simulink model "feng_ct"  (R2016b)
(part 3 of 81)

      | port_label('output', 1, 'q');
      | disp(['Z^-', num2str(latency)]);
  we_delay95 : Subsystem  AncestorBlock=casper_library_delays/pipeline  mask(pipeline){latency=5}
      mask help:
      | An explicitly laid-out delay line to avoid mapping to SRL16s
      | for use in pipelining to help achieve timing closure.
      mask init:
      | pipeline_init(gcb,'latency',latency);
      settings: AttributesFormatString=Latency = %<latency>
      mask Display:
      | port_label('input', 1, 'd');
      | port_label('output', 1, 'q');
      | disp(['Z^-', num2str(latency)]);
  we_delay96 : Subsystem  AncestorBlock=casper_library_delays/pipeline  mask(pipeline){latency=3}
      mask help:
      | An explicitly laid-out delay line to avoid mapping to SRL16s
      | for use in pipelining to help achieve timing closure.
      mask init:
      | pipeline_init(gcb,'latency',latency);
      settings: AttributesFormatString=Latency = %<latency>
      mask Display:
      | port_label('input', 1, 'd');
      | port_label('output', 1, 'q');
      | disp(['Z^-', num2str(latency)]);
  we_delay97 : Subsystem  AncestorBlock=casper_library_delays/pipeline  mask(pipeline){latency=5}
      mask help:
      | An explicitly laid-out delay line to avoid mapping to SRL16s
      | for use in pipelining to help achieve timing closure.
      mask init:
      | pipeline_init(gcb,'latency',latency);
      settings: AttributesFormatString=Latency = %<latency>
      mask Display:
      | port_label('input', 1, 'd');
      | port_label('output', 1, 'q');
      | disp(['Z^-', num2str(latency)]);
  we_delay98 : Subsystem  AncestorBlock=casper_library_delays/pipeline  mask(pipeline){latency=5}
      mask help:
      | An explicitly laid-out delay line to avoid mapping to SRL16s
      | for use in pipelining to help achieve timing closure.
      mask init:
      | pipeline_init(gcb,'latency',latency);
      settings: AttributesFormatString=Latency = %<latency>
      mask Display:
      | port_label('input', 1, 'd');
      | port_label('output', 1, 'q');
      | disp(['Z^-', num2str(latency)]);
  we_delay99 : Subsystem  AncestorBlock=casper_library_delays/pipeline  mask(pipeline){latency=3}
      mask help:
      | An explicitly laid-out delay line to avoid mapping to SRL16s
      | for use in pipelining to help achieve timing closure.
      mask init:
      | pipeline_init(gcb,'latency',latency);
      settings: AttributesFormatString=Latency = %<latency>
      mask Display:
      | port_label('input', 1, 'd');
      | port_label('output', 1, 'q');
      | disp(['Z^-', num2str(latency)]);
  xsg_core_config : Subsystem  Tag=xps:xsg  AncestorBlock=xps_library/XSG_core_config  mask(xsg core config){hw_sys=SKARAB:xc7vx690t, clk_src=sys_clk, clk_rate=238, sample_period=1, synthesis_tool=XST}
      mask prompts: hw_sys "Hardware Platform"; clk_src "User IP Clock source"; clk_rate "User IP Clock Rate (MHz)"; sample_period "Sample Period"; synthesis_tool "Synthesis Tool:"
      mask help:
      | The XSG Core Config block is used to configure the System Generator design
      | for the casper_xps toolflow. Settings here are used to configure the
      | Xilinx System Generator block parameters automatically, and control toolflow
      | script  execution. It needs to be at the top level of all designs being compiled
      | with the casper_xps toolflow.
      mask init:
      | xps_xsg_conf_mask;
      mask Help: eval('xlWeb([getenv(''MLIB_ROOT''), ''\doc\html\sys_xsg_core_config\sys_xsg_core_config.html''])')
      mask TypeOptions hw_sys: ROACH:sx95t | ROACH:lx110t | ROACH2:sx475t | SNAP:xc7k160t | KC705:xc7k325t | SKARAB:xc7vx690t
      mask Callback hw_sys: xps_xsg_conf_callback
      mask TypeOptions clk_src: sys_clk | aux_clk
      mask Callback clk_src: xps_xsg_conf_callback
      mask Callback clk_rate: xps_xsg_conf_callback
      mask TypeOptions synthesis_tool: Leonardo Spectrum | Synplify | Synplify Pro | XST
      mask Display: fprintf(['MSSGE\n', hw_sys]);
  tag scope: cnt_rst=global, ct_chans_per_board=global, ct_chans_per_x=global, ct_chans_per_x_hmc_par=global, ct_chans_per_x_hmc_par_recip=global, ct_chans_per_x_par=global, ct_chans_per_x_recip=global, ct_fake_data_error=global, ct_num_x_boards=global, ct_num_x_boards_recip=global, ct_num_xeng=global, ct_num_xeng_recip=global, ct_rst_err_latch=global, ct_tag_insert_sel=global, ct_tvg_en2=global, ct_tvg_en=global, ct_x_per_board=global, ct_x_per_board_recip=global, obuf_read_gap=global, pktoffset_sel=global, pktstart_sel=global, sys_rst=global, tvgtone_levels=global, tvgtone_p0=global, tvgtone_p1=global, up_timestep_error=global
  wires:
  Constant3/1 -> gbe0/8(rx_overrun_ack)
  Constant4/1 -> gbe0/7(rx_ack)
  [gbe_rst] -> pipeline99/1(d)
  unpack_and_reorder/5(recvd) -> pipeline17/1(d)
  sync_gen/2(dout) -> bus_expand6/1(bus_in)
  sync_gen/3(dvalid) -> impulse_gen0/6(en), impulse_gen1/6(en)
  Slice4/1 -> pipeline16/1(d)
  pipeline16/1(q) -> local_time_lsw/1(out_timestamp_lsw)
  Slice16/1 -> Convert6/1
  pipeline47/1(q) -> local_time_msw/1(out_timestamp_msw)
  Convert6/1 -> pipeline47/1(d)
  [time80_48] -> Slice16/1, Slice4/1
  Concat22/1 -> [ld_val0]
  Concat3/1 -> [ld_val1]
  bus_expand17/1(msb_out2) -> [unpack_recvd0]
  bus_expand17/2(lsb_out1) -> [unpack_recvd1]
  Slice12/1 -> [time80]
  impulse_gen0/3(dvalid) -> [valid80]
  impulse_gen0/1(sync_out) -> [sync80]
  impulse_gen0/2(dout) -> [d80_adc0]
  impulse_gen0/4(misco) -> [time80_48], Slice12/1
  [tvg_adc_en] -> impulse_gen0/1(tvg_en)
  impulse_gen1/1(sync_out) -> Terminator6/1
  impulse_gen1/2(dout) -> [d80_adc1]
  impulse_gen1/3(dvalid) -> Terminator8/1
  impulse_gen1/4(misco) -> [dig_flags]
  [tvg_adc_en] -> impulse_gen1/1(tvg_en)
  impulse0/1(in_offset) -> Slice7/1
  impulse0/2(in_amplitude) -> impulse_gen0/3(impulse_amplitude)
  impulse1/1(in_offset) -> Slice8/1
  impulse1/2(in_amplitude) -> impulse_gen1/3(impulse_amplitude)
  sync_gen/1(sync) -> impulse_gen0/4(sync_in), impulse_gen1/4(sync_in)
  bus_expand6/1(msb_out2) -> impulse_gen0/5(din)
  bus_expand6/2(lsb_out1) -> impulse_gen1/5(din)
  sync_gen/5(misco) -> impulse_gen1/7(misci)
  sync_gen/4(time_out) -> impulse_gen0/7(misci)
  Constant31/1 -> Concat9/2
  [unpack_timestamp] -> Concat9/1
  [up_timestep_error] -> Logical15/1
  [sys_rst] -> Logical15/2
  Logical15/1 -> edge_detect17/1(in)
  edge_detect17/1(out) -> [sys_relock]
  phase0/1(in_initial) -> Reinterpret2/1
  delta_delay0/1(in_delta) -> Reinterpret1/1
  phase0/2(in_delta) -> Reinterpret3/1
  Concat9/1 -> sync_gen/1(time_in)
  [sys_relock] -> sync_gen/5(relock)
  [unpack_dv] -> sync_gen/2(en)
  [unpack_d160] -> sync_gen/3(din)
  Slice7/1 -> impulse_gen0/2(impulse_offset)
  Slice8/1 -> impulse_gen1/2(impulse_offset)
  Reinterpret8/1 -> Concat22/1
  Reinterpret1/1 -> Concat22/2
  Reinterpret2/1 -> Concat22/3
  Reinterpret3/1 -> Concat22/4
  phase1/1(in_initial) -> Reinterpret5/1
  delta_delay1/1(in_delta) -> Reinterpret4/1
  phase1/2(in_delta) -> Reinterpret6/1
  Reinterpret4/1 -> Concat3/2
  Reinterpret5/1 -> Concat3/3
  Reinterpret6/1 -> Concat3/4
  Reinterpret7/1 -> Concat3/1
  delay0/1(in_initial) -> Reinterpret8/1
  delay1/1(in_initial) -> Reinterpret7/1
  trig_time_msw/1(in_msw) -> pipeline28/1(d)
  trig_time_lsw/1(in_lsw) -> pipeline44/1(d)
  Concat13/1 -> Relational10/1
  pipeline28/1(q) -> Concat13/1
  pipeline44/1(q) -> Concat13/2
  [valid80] -> Counter/2
  [sync80] -> Counter/1
  Constant12/1 -> Relational7/2
  Counter/1 -> Relational7/1
  Relational10/1 -> Mux/2
  Relational7/1 -> Mux/3
  [valid80] -> Delay49/1
  Logical12/1 -> Logical14/1
  Logical14/1 -> [adc_snap_trig]
  [adc_snap_arm] -> Logical14/2
  [time80_48] -> Relational10/2
  Delay49/1 -> Logical12/2
  Mux/1 -> Logical12/1
  [adc_snap_trig_source] -> Mux/1
  iptx_base/1(in_reg) -> pipeline105/1(d)
  pipeline105/1(q) -> [tx_ip_base]
  tx_metadata/1(in_porttx) -> pipeline106/1(d)
  tx_metadata/2(in_board_id) -> pipeline107/1(d)
  pipeline106/1(q) -> [tx_port]
  pipeline107/1(q) -> changing_bits2/1
  edge_detect4/1(out) -> pipeline5/1(d)
  control/6(in_cnt_rst) -> edge_detect1/1(in)
  edge_detect1/1(out) -> pipeline14/1(d)
  control/3(in_gbe_rst) -> pipeline6/1(d)
  control/1(in_sys_rst) -> pipeline3/1(d)
  pipeline3/1(q) -> [sys_rst]
  pipeline5/1(q) -> [clr_status]
  pipeline6/1(q) -> [gbe_rst]
  pipeline7/1(q) -> [gbe_txen]
  pipeline13/1(q) -> [tvg_adc_en]
  pipeline14/1(q) -> [cnt_rst]
  control/5(in_tvg_adc) -> pipeline13/1(d)
  edge_detect2/1(out) -> pipeline38/1(d)
  pipeline38/1(q) -> [gbe_cnt_rst]
  control/7(in_gbe_cnt_rst) -> edge_detect2/1(in)
  control/4(in_gbe_txen) -> pipeline7/1(d)
  control/2(in_status_clr) -> edge_detect4/1(in)
  pipeline43/1(q) -> [adc_snap_arm]
  control/8(in_adc_snap_arm) -> pipeline43/1(d)
  control/9(in_adc_snap_trig_select) -> pipeline39/1(d)
  pipeline39/1(q) -> [adc_snap_trig_source]
  pfb/2(dout0) -> [pfb_d144_0]
  pfb/3(dout1) -> [pfb_d144_1]
  [fft_shift] -> pfb/1(shift)
  fft_shift/1(in_fft_shift) -> pipeline4/1(d)
  pfb/5(of) -> [pfb_of]
  pfb/4(dvalid) -> [pfb_dv]
  pfb/1(sync_out) -> [pfb_sync]
  [pfbin_d1] -> pfb/4(din1)
  [pfbin_d0] -> pfb/3(din0)
  [pfbin_sync] -> pfb/2(sync_in)
  [pfbin_dv] -> pfb/5(en)
  tl_fd0/2(enable) -> phase_compensation0/5(load_value)
  tl_fd1/1(value) -> phase_compensation1/4(delay_value)
  tl_fd1/2(enable) -> phase_compensation1/5(load_value)
  tl_fd0/1(value) -> phase_compensation0/4(delay_value)
  [clr_status] -> tl_fd1/1(rst), tl_fd0/1(rst)
  phase_compensation0/1(sync_out) -> [fdfs_sync]
  phase_compensation1/1(sync_out) -> Terminator24/1
  phase_compensation0/2(dout) -> [fdfs_d144_0]
  phase_compensation1/2(dout) -> [fdfs_d144_1]
  phase_compensation0/3(dvalid) -> [fdfs_dv]
  phase_compensation1/3(dvalid) -> Terminator25/1
  [ld_val0] -> tl_fd0/3(load_value)
  [ld_val1] -> tl_fd1/3(load_value)
  bus_expand16/1(msb_out2) -> tl_fd0/5(din)
  tl_fd0/5(dvalid) -> phase_compensation0/3(en)
  tl_fd0/3(sync_out) -> phase_compensation0/1(sync_in)
  tl_fd0/4(dout) -> phase_compensation0/2(din)
  tl_fd1/4(dout) -> phase_compensation1/2(din)
  bus_expand16/2(lsb_out1) -> tl_fd1/5(din)
  Constant29/1 -> Concat2/2
  Concat2/1 -> tl_fd1/2(current_time), tl_fd0/2(current_time)
  [gbe_cnt_rst] -> pipeline31/1(d)
  pipeline31/1(q) -> gbe0/9(debug_rst)
  Counter2/1 -> pipeline29/1(d)
  Constant26/1 -> eq1/2(data_in)
  Constant11/1 -> eq1/3(we)
  Delay53/1 -> quant1/1(sync_in)
  Delay34/1 -> quant1/2(din)
  eq1/1(data_out) -> quant1/4(coeffs)
  Delay50/1 -> quant1/3(en)
  Counter4/1 -> pipeline27/1(d)
  Constant24/1 -> eq0/2(data_in)
  Constant25/1 -> eq0/3(we)
  Delay51/1 -> quant0/1(sync_in)
  Delay2/1 -> quant0/2(din)
  Delay52/1 -> quant0/3(en)
  eq0/1(data_out) -> quant0/4(coeffs)
  quant0/1(sync_out) -> [q_sync]
  quant0/2(dout) -> Delay7/1
  quant0/3(dvalid) -> Delay6/1
  quant0/4(of) -> Delay11/1
  quant1/2(dout) -> Delay12/1
  quant1/1(sync_out) -> Terminator19/1
  quant1/3(dvalid) -> Terminator21/1
  quant1/4(of) -> Delay13/1
  pipeline27/1(q) -> eq0/1(addr)
  pipeline29/1(q) -> eq1/1(addr)
  [fdfs_sync] -> Delay51/1, pipeline42/1(d)
  [fdfs_d144_0] -> Delay2/1
  [fdfs_dv] -> Delay52/1, pipeline41/1(d)
  pipeline41/1(q) -> Counter4/2
  pipeline42/1(q) -> Counter4/1
  pipeline45/1(q) -> Counter2/2
  [fdfs_sync] -> Delay53/1, pipeline48/1(d)
  [fdfs_d144_1] -> Delay34/1
  [fdfs_dv] -> Delay50/1, pipeline45/1(d)
  pipeline48/1(q) -> Counter2/1
  gbe0/13(rx_dest_ip) -> pipeline115/1(d)
  gbe0/14(rx_dest_port) -> pipeline116/1(d)
  [rx_dest_ip] -> pipeline/1(d)
  pipeline/1(q) -> rx_dest_ip/1(out_reg)
  [rx_dest_port] -> pipeline18/1(d)
  pipeline18/1(q) -> rx_dest_port/1(out_reg)
  gbe0/1(led_up) -> pipeline100/1(d)
  [forty_gbe_led_up] -> pipeline19/1(d)
  gbe0/2(led_rx) -> pipeline101/1(d)
  [forty_gbe_led_rx] -> pipeline20/1(d)
  gbe0/3(led_tx) -> pipeline102/1(d)
  [forty_gbe_led_tx] -> pipeline51/1(d)
  gbe0/4(tx_afull) -> pipeline103/1(d)
  gbe0/5(tx_overflow) -> pipeline104/1(d)
  gbe0/12(rx_overrun) -> pipeline114/1(d)
  pipeline19/1(q) -> gbe_status/1(out_led_up)
  pipeline20/1(q) -> gbe_status/2(out_led_rx)
  pipeline51/1(q) -> gbe_status/3(out_led_tx)
  gbe0/8(rx_source_ip) -> pipeline110/1(d)
  gbe0/9(rx_source_port) -> pipeline111/1(d)
  pipeline55/1(q) -> rx_src_ip/1(out_reg)
  pipeline56/1(q) -> rx_src_port/1(out_reg)
  [forty_gbe_rx_src_port] -> pipeline56/1(d)
  [forty_gbe_rx_src_ip] -> pipeline55/1(d)
  gbe0/6(rx_data) -> pipeline108/1(d)
  gbe0/10(rx_end_of_frame) -> pipeline112/1(d)
  gbe0/11(rx_bad_frame) -> pipeline113/1(d)
  pipeline174/1(q) -> time_gen1/5(rd_en)
  pipeline173/1(q) -> time_gen1/4(rd_sync_in)
  pipeline80/1(q) -> [flag_sync]
  pipeline81/1(q) -> [flag_misc]
  pipeline82/1(q) -> [flag_dvalid]
  pipeline83/1(q) -> [flag_time]
  [s256_d] -> pipeline98/1(d)
  [s256_ip] -> pipeline97/1(d)
  [s256_port] -> pipeline96/1(d)
  Logical2/1 -> gbe0/6(tx_end_of_frame)
  [s256_v] -> Logical1/2
  [s256_eof] -> Logical2/2
  Delay1/1 -> Logical1/1, Logical2/1
  [s256_eof] -> Delay1/2
  pipeline96/1(q) -> gbe0/5(tx_dest_port)
  pipeline97/1(q) -> gbe0/4(tx_dest_ip)
  pipeline98/1(q) -> gbe0/2(tx_data)
  pipeline99/1(q) -> gbe0/1(rst)
  [gbe_txen] -> Delay1/1
  pipeline100/1(q) -> [forty_gbe_led_up]
  pipeline101/1(q) -> [forty_gbe_led_rx]
  pipeline102/1(q) -> [forty_gbe_led_tx]
  pipeline103/1(q) -> [forty_gbe_tx_full]
  pipeline104/1(q) -> [forty_gbe_tx_of]
  pipeline108/1(q) -> [forty_gbe_rx_data]
  pipeline110/1(q) -> [forty_gbe_rx_src_ip]
  pipeline111/1(q) -> [forty_gbe_rx_src_port]
  pipeline112/1(q) -> [forty_gbe_rx_eof]
  pipeline113/1(q) -> [forty_gbe_rx_bad]
  pipeline114/1(q) -> [forty_gbe_rx_overrun]
  pipeline115/1(q) -> [rx_dest_ip]
  pipeline116/1(q) -> [rx_dest_port]
  [forty_gbe_rx_data] -> unpack_and_reorder/1(d256)
  [forty_gbe_rx_valid] -> unpack_and_reorder/2(dv256)
  [forty_gbe_rx_eof] -> unpack_and_reorder/3(eof256)
  unpack_and_reorder/6(flags) -> Terminator9/1
  unpack_and_reorder/2(d160) -> pipeline11/1(d)
  unpack_and_reorder/3(dv) -> pipeline12/1(d)
  unpack_and_reorder/4(time) -> pipeline15/1(d)
  unpack_and_reorder/1(sync) -> pipeline10/1(d)
  Inverter1/1 -> Logical6/1
  [unpack_recvd0] -> Inverter1/1
  [unpack_dv] -> Logical6/2
  Inverter2/1 -> Logical7/1
  [unpack_recvd1] -> Inverter2/1
  [unpack_dv] -> Logical7/2
  Logical7/1 -> Logical/2
  Logical6/1 -> Logical/1
  Logical/1 -> [unpack_missing]
  pipeline10/1(q) -> [unpack_sync]
  pipeline11/1(q) -> [unpack_d160]
  pipeline12/1(q) -> [unpack_dv]
  pipeline15/1(q) -> [unpack_timestamp]
  pipeline17/1(q) -> bus_expand17/1(bus_in)
  [clr_status] -> Counter1/1, Subsystem5/1(rst)
  [up_dbg_rst] -> Subsystem4/1(rst)
  [upg_sp_dv] -> Logical3/2
  [upg_sp_eof] -> Logical3/1
  [upg_reo_time] -> Subsystem1/3(time)
  [upg_reo_recv] -> Subsystem1/4(recv)
  [upg_reo_dv] -> Subsystem7/1(dv), Subsystem1/2(dv)
  [up_dbg_rst] -> Subsystem1/1(rst)
  Subsystem1/7(time_change) -> [reo_time_change]
  Logical5/1 -> Subsystem1/7(overflow_err)
  [upg_of80_p1] -> Logical5/2
  [upg_of80_p0] -> Logical5/1
  [upg_sperr_magic] -> Subsystem4/2(in0)
  [upg_sperr_len] -> Subsystem4/5(in3)
  [upg_sperr_hdr] -> Subsystem4/3(in1)
  [upg_sperr_pad] -> Subsystem4/4(in2)
  pipeline175/1(q) -> time_gen1/6(rd_misc_in)
  tl_fd0/7(misco) -> Terminator2/1
  tl_fd0/6(time) -> Terminator3/1
  tl_fd1/6(time) -> Terminator4/1
  tl_fd1/3(sync_out) -> phase_compensation1/1(sync_in)
  tl_fd1/5(dvalid) -> phase_compensation1/3(en)
  tl_fd1/7(misco) -> Terminator5/1
  Constant18/1 -> tl_fd0/7(misci)
  Constant19/1 -> tl_fd1/7(misci)
  Subsystem4/5(out4) -> spead_status/5(out_pkt_cnt)
  Logical3/1 -> Subsystem4/6(in4)
  Constant1/1 -> sync_gen/4(misci)
  time_gen/1(rd_sync_out) -> tl_fd1/4(sync_in), tl_fd0/4(sync_in)
  time_gen/2(rd_dvalid) -> tl_fd1/6(en), tl_fd0/6(en)
  time_gen/3(rd_val_out) -> Concat2/1
  time_gen/4(rd_misc_out) -> bus_expand16/1(bus_in)
  [sync80] -> time_gen/1(wr_sync_in)
  [valid80] -> time_gen/2(wr_en)
  [pfb_sync] -> time_gen/4(rd_sync_in)
  [pfb_dv] -> time_gen/5(rd_en)
  [pfb_d144_1] -> Concat1/2
  [pfb_d144_0] -> Concat1/1
  Concat1/1 -> time_gen/6(rd_misc_in)
  [q_sync] -> time_gen1/1(wr_sync_in)
  [q_dv] -> time_gen1/2(wr_en)
  [time80] -> Slice2/1
  time_gen1/1(rd_sync_out) -> pipeline80/1(d)
  time_gen1/4(rd_misc_out) -> pipeline81/1(d)
  time_gen1/2(rd_dvalid) -> pipeline82/1(d)
  time_gen1/3(rd_val_out) -> pipeline83/1(d)
  [time80] -> time_gen/3(wr_val_in)
  Slice2/1 -> time_gen1/3(wr_val_in)
  pipeline4/1(q) -> [fft_shift]
  Logical1/1 -> gbe0/3(tx_valid)
  pipeline59/1(q) -> [ct_tvg_en]
  control/10(in_ct_tvg_en) -> pipeline59/1(d)
  pipeline52/1(q) -> [up_dbg_rst]
  control/11(in_unpack_debug_reset) -> pipeline52/1(d)
  Subsystem1/8(timestep_err) -> [up_timestep_error]
  Subsystem4/4(out3) -> spead_status/4(out_pkt_len_err_cnt)
  Subsystem4/3(out2) -> spead_status/3(out_pad_err_cnt)
  Subsystem4/2(out1) -> spead_status/2(out_header_err_cnt)
  Subsystem4/1(out0) -> spead_status/1(out_magic_err_cnt)
  [upg_reo_disc] -> Subsystem1/5(discard_err)
  [upg_reo_relock] -> Subsystem1/6(relock_err)
  Subsystem1/1(timestep_err_cnt) -> reorder_status/1(out_timestep_err_cnt)
  Subsystem1/2(recv_err_cnt) -> reorder_status/2(out_receive_err_cnt)
  Subsystem1/3(discard_err_cnt) -> reorder_status/3(out_discard_cnt)
  Subsystem1/4(relock_err_cnt) -> reorder_status/4(out_relock_err_cnt)
  Subsystem1/5(overflow_err_cnt) -> reorder_status/5(out_overflow_err_cnt)
  Subsystem2/1(out0) -> cd_status/1(out_hmc_err_cnt)
  Subsystem2/2(out1) -> cd_status/2(out_pol0_parity_err_cnt)
  Subsystem2/3(out2) -> cd_status/3(out_pol1_parity_err_cnt)
  [hmc_parity_pol0] -> Subsystem2/3(in1)
  [hmc_parity_pol1] -> Subsystem2/4(in2)
  [clr_status] -> Subsystem2/1(rst)
  [hmc_error] -> Subsystem2/2(in0)
  [clr_status] -> Subsystem3/1(rst)
  Slice/1 -> Subsystem3/2(in0)
  [pfb_of] -> Slice/1, Slice6/1
  Slice6/1 -> Subsystem3/3(in1)
  [pfb_sync] -> Subsystem3/4(in2)
  Subsystem3/3(out2) -> pfb_status/3(out_sync_cnt)
  Subsystem5/1(out0) -> quant_status/1(out_pol0_or_cnt)
  Relational/1 -> Subsystem5/2(in0)
  Constant10/1 -> Relational/2
  [q_of0] -> Relational/1
  Relational3/1 -> Subsystem5/3(in1)
  [q_of1] -> Relational3/1
  Constant13/1 -> Relational3/2
  Subsystem5/2(out1) -> quant_status/2(out_pol1_or_cnt)
  Subsystem3/1(out0) -> pfb_status/1(out_pol0_or_err_cnt)
  Subsystem3/2(out1) -> pfb_status/2(out_pol1_or_err_cnt)
  [q_sync] -> hmc_ct/1(in_sync)
  [q_d64_1] -> Concat4/1
  [q_d64_0] -> Concat4/2
  hmc_ct/4(pkt_start) -> [ct_pktstart]
  [ct_tvg_en2] -> Mux1/1
  hmc_ct/1(out_sync) -> [ct_sync]
  hmc_ct/2(out_dv) -> [ct_dv]
  hmc_ct/3(out_d256) -> [ct_d256]
  [ct_dv] -> pipeline86/1(d)
  pipeline87/1(q) -> Mux1/2
  pipeline85/1(q) -> tvg/1(sync), pipeline89/1(d)
  [ct_sync] -> pipeline85/1(d)
  [ct_d256] -> pipeline87/1(d)
  pipeline89/1(q) -> pipeline173/1(d)
  pipeline88/1(q) -> pipeline174/1(d)
  Mux1/1 -> pipeline175/1(d)
  pipeline86/1(q) -> tvg/2(dv), pipeline88/1(d)
  Subsystem1/6(dv_cnt) -> reorder_status/6(out_dv_cnt)
  [flag_dvalid] -> Subsystem13/1(In1)
  Subsystem13/1(Out1) -> time_status/1(out_dv_cnt)
  tvg/1(data256) -> Mux1/3
  [ct_dv] -> Subsystem8/1(In1)
  Subsystem8/1(Out1) -> ct_dv_rate/1(out_reg)
  we_delay49/1(q) -> [ct_tag_insert_sel]
  edge_detect3/1 -> [ct_rst_err_latch]
  we_delay47/1(q) -> edge_detect3/1
  we_delay48/1(q) -> [ct_fake_data_error]
  we_delay13/1(q) -> [ct_tvg_en]
  we_delay50/1(q) -> [ct_tvg_en2]
  Constant2/1 -> ct_control0/5(sim_5)
  Constant21/1 -> ct_control0/4(sim_4)
  Constant20/1 -> ct_control0/3(sim_3)
  Constant22/1 -> ct_control0/2(sim_2)
  Constant15/1 -> ct_control0/1(sim_1)
  ct_control0/1(in_tvg_en) -> we_delay13/1(d)
  ct_control0/2(in_tvg_en2) -> we_delay50/1(d)
  ct_control0/3(in_rst_err_latch) -> we_delay47/1(d)
  ct_control0/4(in_fake_error) -> we_delay48/1(d)
  ct_control0/5(in_tag_insert) -> we_delay49/1(d)
  pipeline75/1(q) -> pipeline62/1(d)
  [gbe_stopmux] -> multimux4/1(select)
  [forty_gbe_tx_of] -> multimux4/2(input1)
  [forty_gbe_tx_full] -> multimux4/3(input2)
  [forty_gbe_tx_err] -> multimux4/4(input3)
  [q_sync] -> edge_detect/1
  edge_detect/1 -> Counter1/2
  Counter1/1 -> quant_status/3(out_sync_cnt)
  [ct_pktstart] -> we_delay1/1(d)
  [ct_dv] -> we_delay2/1(d)
  we_delay1/1(q) -> pktlen_check/1(pkt_start)
  we_delay2/1(q) -> dv_block_check/1(dv), pktlen_check/2(dv)
  pktlen_check/1(error) -> we_delay7/1(d)
  dv_block_check/1(error) -> we_delay29/1(d)
  [cnt_rst] -> Subsystem6/1(rst)
  we_delay7/1(q) -> [ct_pktlen_err], Subsystem6/2(in0)
  we_delay29/1(q) -> [ct_dvblk_err], Subsystem6/3(in1)
  Subsystem6/1(out0) -> ct_dv_err/1(out_pktlen_err_cnt)
  Subsystem6/2(out1) -> ct_dv_err/2(out_dvblock_err_cnt)
  [q_dv] -> qt_block_check/1(dv)
  [cnt_rst] -> Subsystem12/1(rst)
  Subsystem12/1(out0) -> qt_dv_err/1(out_dvblock_err_cnt)
  [pack_dv_err] -> multimux4/5(input4)
  [unpack_dv] -> reo_block_check/1(dv)
  [cnt_rst] -> Subsystem15/1(rst)
  Subsystem15/1(out0) -> reo_dv_err/1(out_dvblock_err_cnt)
  reo_block_check/1(error) -> Subsystem15/2(in0)
  [sync80] -> Mux4/2
  [cd_bypass] -> Mux4/1
  [delay_sync] -> Mux4/3
  [valid80] -> Mux5/2
  [cd_bypass] -> Mux5/1
  [delay_dv] -> Mux5/3
  Mux4/1 -> [pfbin_sync]
  Mux5/1 -> [pfbin_dv]
  [d80_adc0] -> Mux6/2
  [cd_bypass] -> Mux6/1
  [delay_d0] -> Mux6/3
  Mux6/1 -> [pfbin_d0]
  [d80_adc1] -> Mux7/2
  [cd_bypass] -> Mux7/1
  [delay_d1] -> Mux7/3
  Mux7/1 -> [pfbin_d1]
  pipeline57/1(q) -> [cd_bypass]
  control/12(in_cd_bypass) -> pipeline57/1(d)
  Constant7/1 -> [delay_sync]
  Constant23/1 -> [delay_d0]
  Constant27/1 -> [delay_dv]
  Constant37/1 -> [delay_d1]
  Constant40/1 -> [hmc_error]
  Constant39/1 -> [hmc_parity_pol0]
  Constant38/1 -> [hmc_parity_pol1]
  [cnt_rst] -> Subsystem17/1(rst)
  Subsystem17/1(out0) -> ct_dout_err0/1(out_pol_error_cnt)
  Subsystem17/2(out1) -> ct_dout_err0/2(out_word_error_cnt)
  pktlen_check2/1(error) -> [ct_tvg_data_order_err]
  Subsystem17/3(out2) -> ct_dout_err0/3(out_dout_order_err)
  Register2/1 -> Relational20/2
  [ct_dv] -> Relational20/3, Register2/2  "dv"
  Relational20/1 -> pktlen_check2/1(pkt_start)  "newdata"
  Delay9/1 -> pktlen_check2/2(dv)  "dv_del"
  [ct_dv] -> Delay9/1
  Slice35/1 -> Relational20/1, Register2/1
  [cnt_rst] -> Subsystem9/1(rst)
  [ct_bank_error_g0] -> Subsystem9/2(in0)
  [ct_en_sync_error_g0] -> Subsystem9/3(in1)
  [wr_data_final_g0] -> bus_expand5/1(bus_in)
  bus_expand5/1(msb_out16) -> Slice30/1
  bus_expand5/2(out15) -> Slice25/1
  bus_expand5/3(out14) -> Slice13/1
  bus_expand5/4(out13) -> Slice26/1
  bus_expand5/9(out8) -> Slice24/1
  bus_expand5/10(out7) -> Slice14/1
  bus_expand5/11(out6) -> Slice15/1
  bus_expand5/12(out5) -> Slice22/1
  Slice30/1 -> [rawd0_0]
  Slice25/1 -> [rawd1_0]
  Slice13/1 -> [rawd2_0]
  Slice26/1 -> [rawd3_0]
  Slice22/1 -> [rawd7_0]
  Slice15/1 -> [rawd6_0]
  Slice14/1 -> [rawd5_0]
  Slice24/1 -> [rawd4_0]
  [ct_pktlen_err] -> Logical22/1
  [ct_dvblk_err] -> Logical22/2
  Logical22/1 -> multimux1/2(input1)
  [wrrd_stopmux] -> Slice44/1
  [ct_tvg_data_order_err] -> multimux1/3(input2)
  [ct_snap_err_stop] -> Logical22/3
  [rawd1_0] -> data_repeat_error/1(data)
  [wr_en_final_g0] -> data_repeat_error/2(dv)
  data_repeat_error/1(same_error) -> [ct_wrdata_repeat_err0]
  dv4/1 -> Relational19/2
  Relational19/1 -> [ct_wrdata_d4zero_err0]
  [rawd4_0] -> Relational19/1
  [wr_en_final_g0] -> Relational19/3
  [ct_wrdata_repeat_err0] -> Logical25/1, multimux1/4(input3)
  [ct_wrdata_d4zero_err0] -> multimux1/5(input4), Logical25/2
  Logical25/1 -> multimux1/6(input5)
  dv5/1 -> multimux1/7(input6)
  hmc_ct/5(freq_id) -> [ct_pktfreq]
  pipeline54/1(q) -> pipeline60/1(d)
  pipeline60/1(q) -> pipeline61/1(d)
  pipeline61/1(q) -> pipeline75/1(d)
  pipeline62/1(q) -> [flag_pktstart]
  [q_dv] -> hmc_ct/2(in_dv)
  Concat4/1 -> hmc_ct/3(in_d128)
  qt_block_check/1(error) -> Subsystem12/2(in0)
  Delay7/1 -> [q_d64_0]
  Delay6/1 -> [q_dv]
  Delay11/1 -> [q_of0]
  Delay12/1 -> [q_d64_1]
  Delay13/1 -> [q_of1]
  pipeline72/1(q) -> pipeline73/1(d)
  pipeline73/1(q) -> pipeline74/1(d)
  pipeline77/1(q) -> pipeline76/1(d)
  pipeline76/1(q) -> [flag_pktfreq]
  pipeline74/1(q) -> pipeline77/1(d)
  [ct_d256] -> Slice43/1
  Slice43/1 -> Relational21/2
  [ct_pktfreq] -> Relational21/1
  Relational21/1 -> Logical16/2
  [ct_dv] -> Delay19/1
  Delay19/1 -> Logical16/1
  Logical16/1 -> [freq_sync_error]
  [cnt_rst] -> Subsystem16/1(rst)
  [hmc_sync_g] -> multimux1/8(input7)
  [freq_sync_error] -> multimux4/6(input5)
  Slice44/1 -> multimux1/1(select)
  multimux4/1(output) -> [ct_snap_err_stop]
  [cnt_rst] -> Subsystem18/1(rst)
  [sync_hmc_in0] -> Subsystem18/2(in0)
  [q_sync] -> Subsystem19/5(in3)
  [pfb_sync] -> Subsystem19/3(in1)
  [fdfs_sync] -> Subsystem19/4(in2)
  [sync80] -> Subsystem19/2(in0)
  [cnt_rst] -> Subsystem19/1(rst)
  Subsystem19/1(out0) -> sync_ctrs1/1(out_sync80)
  Subsystem19/2(out1) -> sync_ctrs1/2(out_pfb)
  Subsystem19/3(out2) -> sync_ctrs1/3(out_fdfs)
  Subsystem19/4(out3) -> sync_ctrs1/4(out_quant)
  [freq_sync_error] -> Subsystem16/3(in1)
  [rd_go_err_g] -> Subsystem16/2(in0)
  Subsystem16/1(out0) -> ct_status3/1(out_out_go_err)
  Subsystem16/2(out1) -> ct_status3/2(out_freq_sync_err)
  Subsystem7/1(per_sec) -> reorder_status1/1(out_dv_per_sec)
  Constant/1 -> [forty_gbe_tx_err]
  gbe0/7(rx_valid) -> pipeline91/1(d)
  pipeline91/1(q) -> [forty_gbe_rx_valid]
  [cnt_rst] -> Subsystem20/1(rst)
  [ct_en_sync_error_g1] -> Subsystem9/5(in3)
  [ct_bank_error_g1] -> Subsystem9/4(in2)
  Subsystem9/2(out1) -> ct_status0/2(out_err_en_sync0)
  Subsystem9/4(out3) -> ct_status0/4(out_err_en_sync1)
  Subsystem9/1(out0) -> ct_status0/1(out_err_bank0)
  Subsystem9/3(out2) -> ct_status0/3(out_err_bank1)
  [hmc_err_rdrdy_g0] -> Subsystem20/3(in1)
  [hmc_err_wrrdy_g0] -> Subsystem20/2(in0)
  Subsystem20/2(out1) -> ct_status1/2(out_err_wrrdy0)
  Subsystem20/1(out0) -> ct_status1/1(out_err_rdrdy0)
  [wr_data_final_g1] -> bus_expand1/1(bus_in)
  bus_expand1/1(msb_out16) -> Slice29/1
  bus_expand1/2(out15) -> Slice20/1
  bus_expand1/3(out14) -> Slice9/1
  bus_expand1/4(out13) -> Slice21/1
  bus_expand1/9(out8) -> Slice19/1
  bus_expand1/10(out7) -> Slice10/1
  bus_expand1/11(out6) -> Slice17/1
  bus_expand1/12(out5) -> Slice18/1
  Slice29/1 -> [rawd0_1]
  Slice20/1 -> [rawd1_1]
  Slice9/1 -> [rawd2_1]
  Slice21/1 -> [rawd3_1]
  Slice18/1 -> [rawd7_1]
  Slice17/1 -> [rawd6_1]
  Slice10/1 -> [rawd5_1]
  Slice19/1 -> [rawd4_1]
  Subsystem20/4(out3) -> ct_status1/4(out_err_rdrdy1)
  Subsystem20/6(out5) -> ct_status1/6(out_wr_ctr1)
  Subsystem20/5(out4) -> ct_status1/5(out_err_wrrdy1)
  Subsystem20/3(out2) -> ct_status1/3(out_wr_ctr0)
  [wr_en_final_g0] -> Subsystem20/4(in2)
  [hmc_err_wrrdy_g1] -> Subsystem20/5(in3)
  [hmc_err_rdrdy_g1] -> Subsystem20/6(in4)
  [wr_en_final_g1] -> Subsystem20/7(in5)
  [wr_addr_final_g0] -> Slice1/1
  [rd_addr_final_g0] -> Slice31/1
  [wr_addr_raw_g0] -> we_delay24/1(d)
  Slice1/1 -> we_delay33/1(d)
  [rd_arm_final_g0] -> we_delay34/1(d)
  [rd_en_final_g0] -> we_delay35/1(d)
  [rd_addr_raw_final_g0] -> we_delay36/1(d)
  Slice31/1 -> we_delay55/1(d)
  [wr_en_final_g0] -> we_delay21/1(d)
  [hmc_wr_sync_g0] -> we_delay14/1(d)
  [hmc_rd_rdy_g0] -> we_delay11/1(d)
  [hmc_wr_rdy_g0] -> we_delay10/1(d)
  we_delay10/1(q) -> Reinterpret/1
  we_delay11/1(q) -> Reinterpret11/1
  we_delay14/1(q) -> Reinterpret12/1
  we_delay21/1(q) -> Reinterpret13/1
  we_delay24/1(q) -> hmc_readwrite0/5(in_wr_addr_raw)
  we_delay33/1(q) -> hmc_readwrite0/6(in_wr_addr)
  we_delay34/1(q) -> Reinterpret14/1
  we_delay35/1(q) -> Reinterpret15/1
  we_delay56/1(q) -> hmc_readwrite0/7(in_wr_d0)
  [rawd0_0] -> we_delay56/1(d)
  we_delay57/1(q) -> hmc_readwrite0/8(in_wr_d4)
  [rawd4_0] -> we_delay57/1(d)
  we_delay3/1(q) -> Reinterpret18/1
  [ct_bank_error_g0] -> we_delay3/1(d)
  [ct_en_sync_error_g0] -> we_delay4/1(d)
  we_delay4/1(q) -> Reinterpret16/1
  [cthmc_sync_err_g0] -> we_delay5/1(d)
  we_delay5/1(q) -> Reinterpret17/1
  Reinterpret/1 -> hmc_readwrite0/1(in_wr_rdy)
  Reinterpret11/1 -> hmc_readwrite0/2(in_rd_rdy)
  Reinterpret12/1 -> hmc_readwrite0/3(in_wr_sync)
  Reinterpret13/1 -> hmc_readwrite0/4(in_wr_en)
  Reinterpret14/1 -> hmc_readwrite0/9(in_rd_arm)
  Reinterpret15/1 -> hmc_readwrite0/10(in_rd_en)
  Reinterpret16/1 -> hmc_readwrite0/15(in_sync_err0)
  Reinterpret17/1 -> hmc_readwrite0/16(in_sync_err1)
  Reinterpret18/1 -> hmc_readwrite0/14(in_bank_err)
  [rd_tag_final_g0] -> we_delay42/1(d)
  we_delay42/1(q) -> hmc_readwrite0/13(in_rd_tag)
  [hmc_d256_g0] -> Slice23/1
  Slice23/1 -> we_delay51/1(d)
  [hmc_d256_g1] -> Slice27/1
  Slice27/1 -> we_delay44/1(d)
  [hmc_dv_g1] -> Reinterpret32/1
  [hmc_tag_g1] -> we_delay63/1(d)
  [hmc_dv_g0] -> Reinterpret29/1
  [hmc_tag_g0] -> we_delay58/1(d)
  we_delay51/1(q) -> hmc_readwrite1/3(in_d0)
  we_delay58/1(q) -> hmc_readwrite1/5(in_tag0)
  we_delay63/1(q) -> hmc_readwrite1/8(in_tag1)
  we_delay44/1(q) -> hmc_readwrite1/6(in_d1)
  we_delay54/1(q) -> hmc_readwrite1/4(in_dv0)
  we_delay62/1(q) -> hmc_readwrite1/7(in_dv1)
  [hmc_init_done_g0] -> Reinterpret28/1
  [hmc_postokay_g0] -> Reinterpret23/1
  we_delay8/1(q) -> hmc_readwrite1/1(in_post_ok)
  we_delay9/1(q) -> hmc_readwrite1/2(in_init_done)
  [cnt_rst] -> Subsystem21/1(rst)
  [hmc_postokay_g0] -> Inverter/1
  [hmc_init_done_g0] -> Inverter3/1
  [hmc_init_done_g1] -> Inverter5/1
  [hmc_postokay_g1] -> Inverter4/1
  Subsystem21/2(out1) -> ct_status4/2(out_init_err0)
  Subsystem21/4(out3) -> ct_status4/4(out_init_err1)
  Subsystem21/3(out2) -> ct_status4/3(out_post_err1)
  Subsystem21/1(out0) -> ct_status4/1(out_post_err0)
  Inverter/1 -> Subsystem21/2(in0)
  Inverter3/1 -> Subsystem21/3(in1)
  Inverter4/1 -> Subsystem21/4(in2)
  Inverter5/1 -> Subsystem21/5(in3)
  we_delay55/1(q) -> hmc_readwrite0/11(in_rd_addr)
  we_delay36/1(q) -> hmc_readwrite0/12(in_rd_addr_raw)
  [rd_en_final_g1] -> we_delay23/1(d)
  [wr_en_final_g1] -> we_delay16/1(d)
  [hmc_rd_rdy_g1] -> we_delay12/1(d)
  [hmc_wr_rdy_g1] -> we_delay6/1(d)
  we_delay6/1(q) -> Reinterpret19/1
  we_delay12/1(q) -> Reinterpret20/1
  we_delay16/1(q) -> Reinterpret22/1
  we_delay23/1(q) -> Reinterpret24/1
  we_delay18/1(q) -> Reinterpret27/1
  [ct_bank_error_g1] -> we_delay18/1(d)
  [ct_en_sync_error_g1] -> we_delay26/1(d)
  we_delay26/1(q) -> Reinterpret25/1
  [cthmc_sync_err_g1] -> we_delay28/1(d)
  we_delay28/1(q) -> Reinterpret26/1
  [cnt_rst] -> Subsystem22/1(rst)
  [hmc_dv_clash_g] -> Subsystem22/2(in0)
  [hmc_dv_fixed_clash_g] -> Subsystem22/3(in1)
  [hmc_fifo_full_g] -> Subsystem22/4(in2)
  Subsystem22/3(out2) -> ct_status5/3(out_fifo_full_err)
  Subsystem22/1(out0) -> ct_status5/1(out_dv_clash)
  Subsystem22/2(out1) -> ct_status5/2(out_dv_fixed_clash)
  [ct_d256] -> bus_expand2/1(bus_in)
  bus_expand2/8(lsb_out1) -> [ct_d256_0]
  bus_expand2/5(out4) -> [ct_d256_3]
  bus_expand2/4(out5) -> [ct_d256_4]
  bus_expand2/3(out6) -> [ct_d256_5]
  bus_expand2/2(out7) -> [ct_d256_6]
  bus_expand2/1(msb_out8) -> [ct_d256_7]
  bus_expand2/6(out3) -> [ct_d256_2]
  bus_expand2/7(out2) -> [ct_d256_1]
  [ct_d256_0] -> Slice38/1, Slice37/1
  Slice38/1 -> we_delay45/1(d)
  Slice37/1 -> we_delay/1(d)
  [ct_d256_1] -> Slice28/1
  Slice28/1 -> we_delay46/1(d)
  Slice34/1 -> we_delay64/1(d)
  [ct_d256_7] -> Slice34/1
  we_delay45/1(q) -> output0/2(in_d0_1)
  we_delay/1(q) -> output0/1(in_d0_0)
  we_delay46/1(q) -> output0/3(in_d1_0)
  Slice32/1 -> we_delay43/1(d)
  [ct_d256_7] -> Slice32/1
  we_delay43/1(q) -> output1/1(in_d7_1)
  [ct_sync] -> we_delay59/1(d)
  [ct_pktstart] -> we_delay61/1(d)
  [ct_dv] -> we_delay53/1(d)
  we_delay53/1(q) -> output0/5(in_dv)
  we_delay61/1(q) -> output0/7(in_pkt_start)
  we_delay59/1(q) -> output0/6(in_sync)
  we_delay64/1(q) -> output0/4(in_d7_0)
  [ct_pktfreq] -> we_delay65/1(d)
  we_delay65/1(q) -> output1/2(in_pkt_freq)
  [raw_freq_ctr_g] -> Slice50/1, Slice51/1
  Slice51/1 -> we_delay91/1(d)
  Slice50/1 -> we_delay90/1(d)
  [sync_hmc_in1] -> Subsystem18/3(in1)
  [sync_obuf_in] -> Subsystem18/4(in2)
  [sync_obuf_out] -> Subsystem18/5(in3)
  Subsystem18/1(out0) -> sync_ctrs2/1(out_hmc_in0)
  Subsystem18/2(out1) -> sync_ctrs2/2(out_hmc_in1)
  Subsystem18/3(out2) -> sync_ctrs2/3(out_hmc_out)
  Subsystem18/4(out3) -> sync_ctrs2/4(out_obuf_out)
  [cthmc_sync_err_g0] -> Subsystem16/4(in2)
  Subsystem16/3(out2) -> ct_status3/3(out_hmc_sync_error)
  Reinterpret26/1 -> hmc_readwrite0/23(in_sync_err11)
  Reinterpret24/1 -> hmc_readwrite0/20(in_rd_en1)
  Reinterpret22/1 -> hmc_readwrite0/19(in_wr_en1)
  Reinterpret20/1 -> hmc_readwrite0/18(in_rd_rdy1)
  Reinterpret19/1 -> hmc_readwrite0/17(in_wr_rdy1)
  Reinterpret25/1 -> hmc_readwrite0/22(in_sync_err01)
  Reinterpret27/1 -> hmc_readwrite0/21(in_bank_err1)
  Mux10/1 -> hmc_readwrite0/27(arm), hmc_readwrite1/13(arm)
  [hmc_sync_g] -> Reinterpret33/1
  we_delay17/1(q) -> hmc_readwrite1/9(in_sync_in)
  [ct_snap_trigsel] -> we_delay66/1(d)
  [ct_snap_wesel] -> we_delay20/1(d)
  Mux8/1 -> we_delay19/1(d)
  dv1/1 -> Mux9/3
  dv3/1 -> Mux9/2
  [hmc_sync_g] -> Mux10/2, Mux8/2
  we_delay19/1(q) -> hmc_readwrite0/25(trig), hmc_readwrite1/11(trig)
  dv7/1 -> Mux10/3
  [ct_snap_trig] -> Mux8/3
  Reinterpret23/1 -> we_delay8/1(d)
  Reinterpret28/1 -> we_delay9/1(d)
  Reinterpret29/1 -> we_delay54/1(d)
  Reinterpret32/1 -> we_delay62/1(d)
  Reinterpret33/1 -> we_delay17/1(d)
  Mux9/1 -> hmc_readwrite0/24(we), hmc_readwrite1/10(we)
  [ct_snap_trigsel] -> we_delay95/1(d)
  [ct_snap_wesel] -> we_delay94/1(d)
  [ct_dv] -> Mux17/3
  dv13/1 -> Mux17/2
  [ct_sync] -> Mux3/2, Mux2/2
  dv14/1 -> Mux2/3
  [ct_snap_trig] -> Mux3/3
  Mux2/1 -> output2/6(arm), output0/11(arm), output1/8(arm)
  Mux3/1 -> output0/9(trig), output1/6(trig), output2/4(trig)
  Mux17/1 -> output0/8(we), output1/5(we), output2/3(we)
  we_delay90/1(q) -> output2/1(in_pkt_ctr_msb)
  we_delay91/1(q) -> output2/2(in_pkt_ctr_lsb)
  [ct_snap_trigsel] -> we_delay71/1(d)
  we_delay20/1(q) -> Mux9/1
  we_delay66/1(q) -> Mux8/1
  we_delay71/1(q) -> Mux10/1
  we_delay94/1(q) -> Mux17/1
  we_delay95/1(q) -> Mux3/1
  [ct_sync] -> Reinterpret39/1
  [ct_dv] -> Reinterpret38/1
  we_delay87/1(q) -> output1/3(in_dv)
  we_delay96/1(q) -> output1/4(in_sync)
  Reinterpret38/1 -> we_delay87/1(d)
  Reinterpret39/1 -> we_delay96/1(d)
  [freq_sync_error] -> output0/10(stop)
  [freq_sync_error] -> output1/7(stop)
  [freq_sync_error] -> output2/5(stop)
  dv12/1 -> Mux18/2
  Mux18/1 -> output2/7(circ), output1/9(circ), output0/12(circ)
  dv15/1 -> Mux18/3
  [ct_snap_trigsel] -> we_delay97/1(d)
  we_delay97/1(q) -> Mux2/1
  [ct_snap_trigsel] -> we_delay98/1(d)
  we_delay98/1(q) -> Mux18/1
  dv20/1 -> Mux21/2
  dv21/1 -> Mux21/3
  [ct_snap_trigsel] -> we_delay103/1(d)
  we_delay103/1(q) -> Mux21/1
  Mux21/1 -> hmc_readwrite0/28(circ), hmc_readwrite1/14(circ)
  [freq_sync_error] -> hmc_readwrite1/12(stop)
  [freq_sync_error] -> hmc_readwrite0/26(stop)
  [s256_d] -> Slice33/1, Slice11/1
  Slice11/1 -> we_delay116/1(d)
  Slice33/1 -> we_delay117/1(d)
  [s256_v] -> we_delay118/1(d)
  [s256_eof] -> we_delay119/1(d)
  [s256_of] -> we_delay120/1(d)
  [s256_ip] -> we_delay121/1(d)
  [s256_port] -> we_delay122/1(d)
  we_delay116/1(q) -> gbe_in0/1(in_d_msb)
  we_delay117/1(q) -> gbe_in1/1(in_d_lsb)
  we_delay118/1(q) -> gbe_in2/7(we), gbe_in2/1(in_dv), gbe_in1/2(we), gbe_in0/2(we)
  we_delay119/1(q) -> gbe_in2/2(in_eof)
  we_delay120/1(q) -> gbe_in2/3(in_of)
  we_delay121/1(q) -> gbe_in2/4(in_ip)
  we_delay122/1(q) -> gbe_in2/5(in_port)
  [ct_snap_trig] -> gbe_in2/8(trig), gbe_in1/3(trig), gbe_in0/3(trig)
  pipeline30/1(q) -> pipeline32/1(d)
  pipeline32/1(q) -> pipeline33/1(d)
  pipeline33/1(q) -> pipeline34/1(d)
  pipeline34/1(q) -> pipeline35/1(d)
  pipeline35/1(q) -> [flag_pktxindex]
  [s256_pktxindex] -> we_delay123/1(d)
  we_delay123/1(q) -> gbe_in2/6(in_xindex)
  hmc_ct/6(x_index) -> [ct_pkt_x_index]
  hmc_ct/7(x_pkt_index) -> [ct_pkt_x_offset]
  pipeline40/1(q) -> pipeline46/1(d)
  pipeline46/1(q) -> pipeline49/1(d)
  pipeline49/1(q) -> pipeline50/1(d)
  pipeline50/1(q) -> pipeline58/1(d)
  pipeline58/1(q) -> [flag_pktxoffset]
  [flag_sync] -> packetiser/1(sync_in)
  [flag_dvalid] -> packetiser/2(en)
  [flag_pktstart] -> packetiser/5(pkt_start)
  [flag_pktxindex] -> packetiser/6(pkt_x_index)
  [flag_pktxoffset] -> packetiser/7(pkt_x_offset)
  [tx_ip_base] -> packetiser/9(base_ip)
  [tx_port] -> packetiser/10(base_port)
  Constant46/1 -> concat1/2
  [flag_time] -> concat1/1
  [flag_misc] -> packetiser/3(din)
  concat1/1 -> [pack_sync_time], packetiser/4(timestamp)
  pipeline65/1(q) -> [s256_d]
  pipeline66/1(q) -> [s256_v]
  pipeline67/1(q) -> [s256_eof]
  pipeline68/1(q) -> [s256_of]
  pipeline69/1(q) -> [s256_ip]
  pipeline70/1(q) -> [s256_port]
  pipeline71/1(q) -> Terminator7/1
  packetiser/1(dout) -> pipeline65/1(d)
  packetiser/2(dvalid) -> pipeline66/1(d)
  packetiser/3(eof) -> pipeline67/1(d)
  packetiser/4(overflow) -> pipeline68/1(d)
  packetiser/5(destination_ip) -> pipeline69/1(d)
  packetiser/6(destination_port) -> pipeline70/1(d)
  packetiser/7(sync) -> pipeline71/1(d)
  [flag_pktfreq] -> pipeline36/1(d)
  pipeline78/1(q) -> [s256_pktfreq]
  pipeline36/1(q) -> pipeline78/1(d)
  [flag_pktxindex] -> pipeline63/1(d)
  pipeline63/1(q) -> pipeline37/1(d)
  pipeline37/1(q) -> [s256_pktxindex]
  [flag_pktxoffset] -> pipeline79/1(d)
  pipeline79/1(q) -> pipeline64/1(d)
  pipeline64/1(q) -> [s256_pktxoffset]
  [tx_board_id] -> packetiser/8(board_id)
  changing_bits2/1 -> [tx_board_id]
  [ct_pkt_x_index] -> pipeline30/1(d)
  [ct_pkt_x_offset] -> pipeline40/1(d)
  [ct_pktfreq] -> pipeline72/1(d)
  [ct_pktstart] -> pipeline54/1(d)
  [flag_pktstart] -> pipeline90/1(d)
  pipeline90/1(q) -> pipeline109/1(d)
  pipeline109/1(q) -> [s256_pktstart]
  we_delay41/1(q) -> [ct_num_xeng]
  we_delay112/1(q) -> [ct_num_xeng_recip]  "NUM_X_RECIP"
  ct_control1/2(in_num_x_recip) -> we_delay112/1(d)
  ct_control1/1(in_num_x) -> we_delay41/1(d)
  we_delay114/1(q) -> [ct_x_per_board]
  ct_control1/3(in_x_per_board) -> we_delay114/1(d)
  we_delay39/1(q) -> [ct_chans_per_x], Slice3/1  "PER_X"
  we_delay113/1(q) -> [ct_chans_per_board]
  ct_control2/1(in_chans_per_x) -> we_delay39/1(d)
  ct_control2/2(in_chans_per_board) -> we_delay113/1(d)
  Slice3/1 -> Slice39/1, [ct_chans_per_x_par]  "PARPAR"
  we_delay115/1(q) -> [ct_x_per_board_recip]
  ct_control1/4(in_x_per_board_recip) -> we_delay115/1(d)
  we_delay38/1(q) -> [ct_num_x_boards]
  ct_control3/1(in_num_x_boards) -> we_delay38/1(d)
  we_delay37/1(q) -> [ct_num_x_boards_recip]
  ct_control3/2(in_num_x_boards_recip) -> we_delay37/1(d)
  ct_control3/3(in_chans_per_x_recip) -> we_delay124/1(d)
  we_delay124/1(q) -> Reinterpret40/1, [ct_chans_per_x_recip]
  Slice39/1 -> [ct_chans_per_x_hmc_par]  "per_x_hmc"
  Reinterpret40/1 -> [ct_chans_per_x_hmc_par_recip]
  Constant49/1 -> ct_control1/1(sim_1)
  Constant53/1 -> ct_control1/2(sim_2)
  Constant9/1 -> ct_control1/3(sim_3)
  Constant28/1 -> ct_control2/1(sim_1)
  Constant50/1 -> ct_control2/2(sim_2)
  Constant54/1 -> ct_control1/4(sim_4)
  Constant8/1 -> ct_control3/1(sim_1)
  Constant14/1 -> ct_control3/2(sim_2)
  Constant44/1 -> ct_control3/3(sim_3)
  [time80_48] -> Subsystem/1(In1)
  [q_sync] -> Subsystem/2(In2)
  [q_dv] -> Subsystem/3(In3)
  Subsystem/1(Out1) -> ct_sync_time_msw/1(out_reg)
  Subsystem/2(Out2) -> ct_sync_time_lsw/1(out_reg)
  tvg_tone_levels/2(in_p0i) -> bus_create/2(in2)
  tvg_tone_levels/3(in_p1r) -> bus_create/3(in3)
  tvg_tone_levels/4(in_p1i) -> bus_create/4(in4)
  tvg_tone_levels/1(in_p0r) -> bus_create/1(in1)
  tvg_tone_targets/1(in_p0) -> [tvgtone_p0]
  tvg_tone_targets/2(in_p1) -> [tvgtone_p1]
  Constant5/1 -> tvg_tone_targets/1(sim_1)
  Constant6/1 -> tvg_tone_targets/2(sim_2)
  Constant34/1 -> tvg_tone_levels/4(sim_4)
  Constant16/1 -> tvg_tone_levels/1(sim_1)
  Constant33/1 -> tvg_tone_levels/3(sim_3)
  Constant17/1 -> tvg_tone_levels/2(sim_2)
  bus_create/1(bus_out) -> [tvgtone_levels]
  pipeline1/1(q) -> [gbe_stopmux]
  pipeline21/1(q) -> [outfreq_stopmux]
  ct_debug/6(in_outfreq_stopmux) -> pipeline21/1(d)
  pipeline22/1(q) -> [out_stopmux]
  ct_debug/5(in_out_stopmux) -> pipeline22/1(d)
  ct_debug/7(in_gbe_stopmux) -> pipeline1/1(d)
  pipeline23/1(q) -> [wrrd_stopmux]
  ct_debug/3(in_wrrd_stopmux) -> pipeline23/1(d)
  pipeline24/1(q) -> [in_stopmux]
  ct_debug/1(in_in_stopmux) -> pipeline24/1(d)
  pipeline25/1(q) -> [ct_snap_arm]
  pipeline26/1(q) -> edge_detect5/1
  ct_debug/9(in_snap_trig) -> pipeline26/1(d)
  ct_debug/8(in_snap_arm) -> pipeline25/1(d)
  edge_detect5/1 -> [ct_snap_trig]
  ct_debug/2(in_in_trigmux) -> pipeline53/1(d)
  pipeline53/1(q) -> [in_trigmux]
  ct_debug/4(in_obuf_stopmux) -> pipeline92/1(d)
  pipeline92/1(q) -> [obuf_stopmux]
  ct_debug/10(in_snap_wesel) -> pipeline2/1(d)
  pipeline2/1(q) -> [ct_snap_wesel]
  pipeline8/1(q) -> [ct_snap_trigsel]
  ct_debug/11(in_snap_trigsel) -> pipeline8/1(d)
  pipeline9/1(q) -> [ct_snap_circsel]
  ct_debug/12(in_snap_circsel) -> pipeline9/1(d)
  [s256_v] -> Subsystem11/1(In1)
  Subsystem11/1(Out1) -> pack_status/1(out_dv_rate)
  [s256_v] -> pack_block_check/1(dv)
  [cnt_rst] -> Subsystem14/1(rst)
  Subsystem14/1(out0) -> pack_dv_err/1(out_dvblock_err_cnt)
  pack_block_check/1(error) -> [pack_dv_err], Subsystem14/2(in0)
  [pack_sync_time] -> Subsystem23/1(time)
  [flag_sync] -> Subsystem23/2(In2)
  [flag_dvalid] -> Subsystem23/3(In3)
  Subsystem23/1(Out1) -> pack_sync_time_msw/1(out_reg)
  Subsystem23/2(Out2) -> pack_sync_time_lsw/1(out_reg)
  gbeout_snap_config/1(in_snap_arm) -> pipeline93/1(d)
  gbeout_snap_config/2(in_pktstart_mux) -> pipeline94/1(d)
  gbeout_snap_config/3(in_pktoffset_mux) -> pipeline95/1(d)
  gbeout_snap_config/4(in_pack_mux) -> pipeline117/1(d)
  pipeline93/1(q) -> [gbeout_snap_arm]
  pipeline94/1(q) -> [pktstart_sel]
  pipeline95/1(q) -> [pktoffset_sel]
  pipeline117/1(q) -> [pack_mux]
  pipeline84/1(q) -> [gbeout_snap_wemux]
  gbeout_snap_config/5(in_we_mux) -> pipeline84/1(d)
  we_delay126/1(q) -> [obuf_read_gap]
  ct_control0/6(in_obuf_read_gap) -> we_delay126/1(d)
  [cnt_rst] -> Subsystem10/1(rst)
  [obuf_ct_addr_err_g] -> Subsystem10/2(in0)
  Subsystem10/1(out0) -> ct_status2/1(out_addr_err0_cnt)
  Subsystem10/2(out1) -> ct_status2/2(out_sync_cnt)
  [ct_sync] -> Subsystem10/3(in1)
  [obuf_in_tag_g] -> we_delay31/1(d)
  [obuf_in_d0_g] -> we_delay30/1(d)
  [obuf_wr_addr_g] -> we_delay40/1(d)
  [obuf_in_sync_g] -> Reinterpret9/1
  [obuf_in_dv_g] -> Reinterpret10/1
  [obuf_wr_en_g] -> Reinterpret21/1
  [obuf_rd_en_g] -> Reinterpret30/1
  [obuf_rd_addr_g] -> we_delay67/1(d)
  [obuf_rd_mux_sel_g] -> we_delay70/1(d)
  [obuf_rd_go_g] -> Reinterpret31/1
  [obuf_rd_done_g] -> Reinterpret34/1
  [obuf_rd_busy_g] -> Reinterpret35/1
  [obuf_rd_d0_0_g] -> we_delay76/1(d)
  [obuf_rd_d7_0_g] -> we_delay83/1(d)
  [obuf_rd_d1_0_g] -> we_delay77/1(d)
  [obuf_rd_d2_0_g] -> we_delay78/1(d)
  [obuf_rd_d3_0_g] -> we_delay79/1(d)
  [obuf_rd_d4_0_g] -> we_delay80/1(d)
  [obuf_rd_d5_0_g] -> we_delay81/1(d)
  [obuf_rd_d6_0_g] -> we_delay82/1(d)
  [ct_snap_trigsel] -> we_delay93/1(d)
  [ct_snap_wesel] -> we_delay92/1(d)
  dv2/1 -> Mux13/3
  dv6/1 -> Mux13/2
  [obuf_in_sync_g] -> Mux11/2, Mux12/2
  dv8/1 -> Mux11/3
  [ct_snap_trig] -> Mux12/3
  Reinterpret9/1 -> we_delay32/1(d)
  Reinterpret10/1 -> we_delay60/1(d)
  Reinterpret21/1 -> we_delay52/1(d)
  Reinterpret30/1 -> we_delay68/1(d)
  Reinterpret31/1 -> we_delay69/1(d)
  Reinterpret34/1 -> we_delay72/1(d)
  Reinterpret35/1 -> we_delay73/1(d)
  we_delay72/1(q) -> obuf0/12(in_rd_done)
  we_delay73/1(q) -> obuf0/13(in_rd_busy)
  we_delay60/1(q) -> obuf0/5(in_in_dv)
  we_delay31/1(q) -> obuf0/1(in_in_tag)
  we_delay52/1(q) -> obuf0/7(in_wr_en)
  we_delay70/1(q) -> obuf0/10(in_rd_mux)
  we_delay32/1(q) -> obuf0/4(in_in_sync)
  we_delay68/1(q) -> obuf0/8(in_rd_en)
  we_delay30/1(q) -> obuf0/2(in_in_d0)
  we_delay69/1(q) -> obuf0/11(in_rd_go)
  we_delay67/1(q) -> obuf0/9(in_rd_addr)
  we_delay40/1(q) -> obuf0/3(in_wr_addr)
  Mux11/1 -> obuf0/17(arm), obuf1/12(arm)
  we_delay74/1(q) -> obuf0/15(trig), obuf1/10(trig)
  we_delay81/1(q) -> obuf2/6(in_d5)
  we_delay83/1(q) -> obuf2/8(in_d7)
  we_delay78/1(q) -> obuf2/3(in_d2)
  we_delay76/1(q) -> obuf2/1(in_d0)
  we_delay82/1(q) -> obuf2/7(in_d6)
  Mux12/1 -> we_delay74/1(d)
  Mux13/1 -> obuf1/9(we), obuf0/14(we)
  [ct_snap_trigsel] -> we_delay89/1(d)
  [ct_snap_wesel] -> we_delay88/1(d)
  dv9/1 -> Mux16/3
  dv10/1 -> Mux16/2
  [obuf_rd_sync_g] -> Mux14/2, Mux15/2
  dv11/1 -> Mux14/3
  [ct_snap_trig] -> Mux15/3
  Mux15/1 -> we_delay86/1(d)
  we_delay86/1(q) -> obuf3/7(trig), obuf2/10(trig)
  Mux14/1 -> obuf3/9(arm), obuf2/12(arm)
  Mux16/1 -> obuf3/6(we), obuf2/9(we)
  we_delay88/1(q) -> Mux16/1
  we_delay89/1(q) -> Mux15/1
  we_delay92/1(q) -> Mux13/1
  we_delay93/1(q) -> Mux12/1
  [ct_snap_circsel] -> we_delay99/1(d)
  we_delay99/1(q) -> Mux19/1
  [obuf_err_stop] -> obuf3/8(stop), obuf2/11(stop)
  [ct_snap_circsel] -> we_delay100/1(d)
  we_delay100/1(q) -> Mux20/1
  Mux20/1 -> obuf3/10(circ), obuf2/13(circ)
  [ct_snap_trigsel] -> we_delay101/1(d)
  we_delay101/1(q) -> Mux14/1
  [ct_snap_trigsel] -> we_delay102/1(d)
  we_delay102/1(q) -> Mux11/1
  Mux19/1 -> obuf1/13(circ), obuf0/18(circ)
  [obuf_err_stop] -> obuf0/16(stop), obuf1/11(stop)
  [obuf_wr_d0_g] -> we_delay104/1(d)
  [obuf_wr_d1_g] -> we_delay105/1(d)
  [obuf_wr_d2_g] -> we_delay106/1(d)
  [obuf_wr_d3_g] -> we_delay107/1(d)
  [obuf_wr_d4_g] -> we_delay108/1(d)
  [obuf_wr_d5_g] -> we_delay109/1(d)
  [obuf_wr_d6_g] -> we_delay110/1(d)
  we_delay106/1(q) -> obuf1/3(in_wr_d2)
  we_delay104/1(q) -> obuf1/1(in_wr_d0)
  we_delay105/1(q) -> obuf1/2(in_wr_d1)
  we_delay109/1(q) -> obuf1/6(in_wr_d5)
  we_delay110/1(q) -> obuf1/7(in_wr_d6)
  we_delay107/1(q) -> obuf1/4(in_wr_d3)
  we_delay108/1(q) -> obuf1/5(in_wr_d4)
  we_delay77/1(q) -> obuf2/2(in_d1)
  we_delay79/1(q) -> obuf2/4(in_d3)
  we_delay80/1(q) -> obuf2/5(in_d4)
  [obuf_dv_g] -> Reinterpret42/1
  [obuf_mux_g] -> we_delay25/1(d)
  Reinterpret42/1 -> we_delay22/1(d)
  we_delay22/1(q) -> obuf3/2(in_dv)
  we_delay25/1(q) -> obuf3/3(in_mux)
  [obuf_rd_addr_out_g] -> we_delay27/1(d)
  we_delay27/1(q) -> obuf3/4(in_rd_addr_out)
  [obuf_ct_addr_err_g] -> Logical4/1
  Logical4/1 -> [obuf_err_stop]
  [obuf_rd_sync_g] -> Reinterpret36/1
  Reinterpret36/1 -> we_delay15/1(d)
  we_delay15/1(q) -> obuf3/1(in_sync)
  [obuf_premux_freq_ctr_g] -> we_delay84/1(d)
  we_delay84/1(q) -> obuf3/5(in_premux_freq)
  Slice5/1 -> we_delay130/1(d), Register/1
  we_delay85/1(q) -> Register/2
  [ct_pktstart] -> we_delay85/1(d)
  Relational22/1 -> Logical8/1
  [ct_dv] -> we_delay131/1(d)
  we_delay131/1(q) -> Logical8/2
  Logical8/1 -> [ct_tvg_data_match_err]  "MATCH_ERROR"
  Register/1 -> Relational22/2  "FIRST"
  we_delay130/1(q) -> Relational22/1
  Subsystem17/4(out3) -> ct_dout_err0/4(out_match_errpr)
  [ct_tvg_data_match_err] -> Subsystem17/5(in3)
  [ct_tvg_data_order_err] -> Subsystem17/4(in2)
  [ct_dv] -> check_ct_data_out/1(in_dv)
  [ct_d256] -> check_ct_data_out/2(in_d256)
  check_ct_data_out/1(ct_out_data_error) -> [ct_tvg_data_err]
  check_ct_data_out/2(pol_error) -> Subsystem17/2(in0)
  check_ct_data_out/3(word_error) -> Subsystem17/3(in1)
  [ct_d256] -> Slice35/1
  [ct_d256] -> Slice5/1
  Constant30/1 -> ct_control0/6(sim_6)
  [freq_sync_error] -> Logical4/2
  dv19/1 -> Mux20/2
  dv18/1 -> Mux20/3
  dv16/1 -> Mux19/3
  dv17/1 -> Mux19/2
  we_delay111/1(q) -> obuf1/8(in_wr_d7)
  [obuf_wr_d7_g] -> we_delay111/1(d)
  [obuf_proc_sync_g] -> Reinterpret37/1
  Reinterpret37/1 -> we_delay75/1(d)
  we_delay75/1(q) -> obuf0/6(in_proc_sync)
